simulink model "qt8"  (R2014a)
settings: Solver=ode23tb  StartTime=0.0  StopTime=3  RelTol=1e-3
libraries: powerlib x16, powerlib_meascontrol x1
settings Model: Creator=fn  LastModifiedBy=Administrator

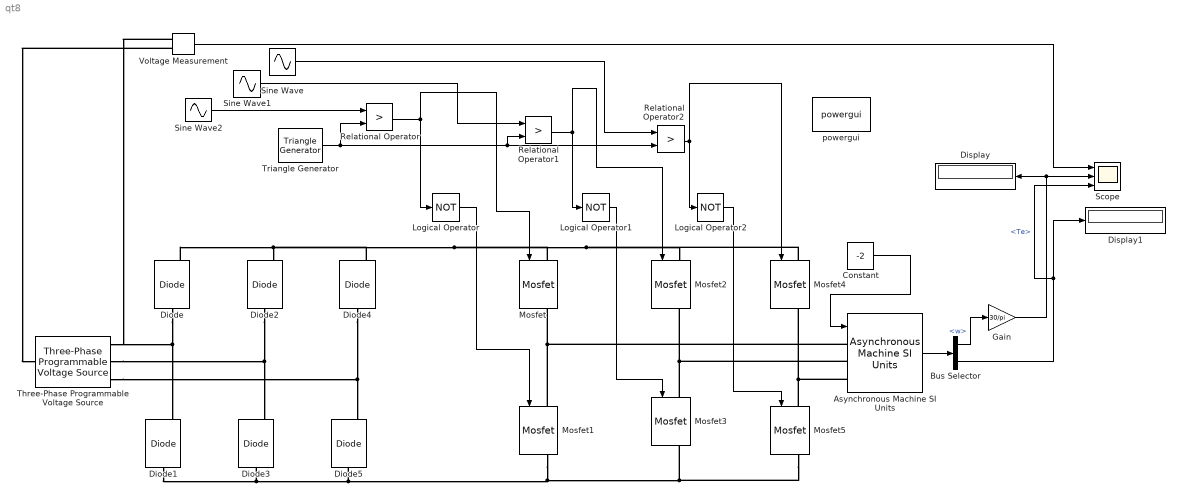
== system qt8 ==
  Asynchronous Machine SI Units : powerlib/Machines/Asynchronous Machine SI Units  PresetModel=No  MechanicalLoad=Torque Tm  ShowDetailedParameters=on  RotorType=Squirrel-cage  ReferenceFrame=Stationary  Units=SI  MeasurementBus=on  NominalParameters=[ 3*746, 220, 60 ]  Stator="[ 0.835  1*2.0e-3 ]"  Rotor="[ 1.016  2.0e-3 ]"  Cage1=[ 0.022 0.226/377]  Cage2=[ 0.022 0.226/377]  Lm=90.31e-3  Mechanical="[ 0.159  0 2]"  PolePairs=2  InitialConditions=[1 0 0 0 0 0 0 0]  SimulateSaturation=off  Saturation=[14.03593122, 27.81365428, 53.79336849, 72.68890987, 97.98006896, 148.6815601, 215.7428561, 302.9841135, 420.4778367 ; 230, 322, 414, 460, 506, 552, 598, 644, 690]  LoadFlowParameters=1492000  TsPowergui=0  TsBlock=-1  IterativeModel=Trapezoidal non iterative  Pmec=0
  Bus Selector : BusSelector  OutputSignals=w,Te
  Constant : Constant  Value=-2
  Diode{,1..5} (6 alike) : powerlib/Power Electronics/Diode  Ron=0.001  Lon=0  Vf=0.8  IC=0  UseSnubber=off  Rs=500  Cs=250e-9  Measurements=on
  Display : Display
  Display1 : Display
  Gain : Gain  Gain=30/pi
  Logical Operator : Logic  Operator=NOT  AllPortsSameDT=off  OutDataTypeStr=boolean
  Logical Operator1 : Logic  Operator=NOT  AllPortsSameDT=off  OutDataTypeStr=boolean
  Logical Operator2 : Logic  Operator=NOT  AllPortsSameDT=off  OutDataTypeStr=boolean
  Mosfet{,1..5} (6 alike) : powerlib/Power Electronics/Mosfet  Ron=0.1  Lon=0  Rd=0.01  Vfd=0  IC=0  Rs=1e5  Cs=inf  Measurements=on
  Relational Operator : RelationalOperator  Operator=>  OutDataTypeStr=boolean
  Relational Operator1 : RelationalOperator  Operator=>  OutDataTypeStr=boolean
  Relational Operator2 : RelationalOperator  Operator=>  OutDataTypeStr=boolean
  Scope : Scope  NumInputPorts=3
      settings: YMin=-200~-100~-5  YMax=200~1500~55
  Sine Wave : Sin  Amplitude=0.8  Frequency=2*pi*30  SampleTime=0
  Sine Wave1 : Sin  Amplitude=0.8  Frequency=2*pi*30  Phase=2/3*pi  SampleTime=0
  Sine Wave2 : Sin  Amplitude=0.8  Frequency=2*pi*30  Phase=-2/3*pi  SampleTime=0
  Three-Phase Programmable Voltage Source : powerlib/Electrical Sources/Three-Phase Programmable Voltage Source  PositiveSequence="[220  0 50]"  VariationEntity=None  VariationType=Table of time-amplitude pairs  VariationTypeAlt=Step  VariationStep=0.5  VariationRate=10  VariationMagnitude=0.3  VariationFrequency=2  VariationTiming=[1 2]  VariationPhaseA=off  Amplitudes=[1 0.8 1.2 1.0]  TimeValues=[0 0.1 0.15 0.2]  HarmonicGeneration=off  HarmonicA=[3 0.2 -25 0]  HarmonicB=[2 0.15 35 2]  Timing="[0.05  3]"  BusType=swing  Pref=0  Qref=0  Qmin=-inf  Qmax=inf
  Triangle Generator : powerlib_meascontrol/Pulse & Signal Generators/Triangle Generator  Freq=1e3  Phase=90  Ts=0
  Voltage Measurement : powerlib/Measurements/Voltage Measurement  PhasorSimulation=off  OutputType=Complex  PSBequivalent=0
  powergui : powerlib/powergui  Priority=1  SimulationMode=Continuous  SolverType=Tustin  SampleTime=50e-6  frequency=60  SPID=off  DisableSnubberDevices=off  DisableRonSwitches=off  DisableVfSwitches=off  SwTol=0  Interpol=off  DisplayEquations=off  Ts=0  methode=off  frequencyindice=50  Pbase=100e6  ErrMax=1e-4  Iterations=50  UnitsV=kV  UnitsW=MW  FunctionMessages=off  echomessages=off  HookPort=off  EnableUseOfTLC=off  x0status=blocks  RestoreLinks=warning  ResistiveCurrentMeasurement=off  Frange=[0:2:500]  Ylog=off  Xlog=on  ShowGrid=off  save=off  variable=ZData  structure=0  ZoomFFT=off  StartTime=0.0  cycles=1  DisplayStyle=1  fundamental=60  FreqAxis=off  MaxFrequency=1000  frequencyindicesteady=1  RmsSteady=1  display=off
  wires:
  Constant/1 -> Asynchronous Machine SI Units/1
  Relational Operator/1 -> Logical Operator/1, Mosfet/1
  Asynchronous Machine SI Units/1 -> Bus Selector/1
  Voltage Measurement/1 -> Scope/1
  Logical Operator/1 -> Mosfet1/1
  Logical Operator2/1 -> Mosfet5/1
  Logical Operator1/1 -> Mosfet3/1
  Relational Operator1/1 -> Mosfet2/1, Logical Operator1/1
  Relational Operator2/1 -> Mosfet4/1, Logical Operator2/1
  Triangle Generator/1 -> Relational Operator1/2, Relational Operator2/2, Relational Operator/2
  Sine Wave/1 -> Relational Operator2/1
  Sine Wave1/1 -> Relational Operator1/1
  Sine Wave2/1 -> Relational Operator/1
  Bus Selector/2 -> Display1/1, Scope/3  "<Te>"
  Bus Selector/1 -> Gain/1  "<w>"
  Gain/1 -> Scope/2, Display/1
  connections:
  Diode/LConn1 -- Voltage Measurement/LConn1 -- Three-Phase Programmable Voltage Source/RConn1 -- Diode1/RConn1
  Diode2/LConn1 -- Three-Phase Programmable Voltage Source/RConn2 -- Diode3/RConn1
  Diode4/LConn1 -- Diode5/RConn1 -- Three-Phase Programmable Voltage Source/RConn3
  Mosfet3/LConn1 -- Asynchronous Machine SI Units/LConn2 -- Mosfet2/RConn1
  Mosfet5/LConn1 -- Asynchronous Machine SI Units/LConn3 -- Mosfet4/RConn1
  Mosfet1/LConn1 -- Asynchronous Machine SI Units/LConn1 -- Mosfet/RConn1
  Voltage Measurement/LConn2 -- Three-Phase Programmable Voltage Source/LConn1
  Diode/RConn1 -- Mosfet4/LConn1 -- Mosfet2/LConn1 -- Mosfet/LConn1 -- Diode4/RConn1 -- Diode2/RConn1
  Diode1/LConn1 -- Diode3/LConn1 -- Mosfet5/RConn1 -- Mosfet3/RConn1 -- Mosfet1/RConn1 -- Diode5/LConn1
